simulink model "mod3tb_CIFF_CRFF_1bit"  (Simulink 7.9)
settings: Solver=VariableStepDiscrete  StartTime=0.0  StopTime=simu.trantime  RelTol=1e-3
undefined symbols (not defined in the file): a, b, c, Fs, g, mod
libraries: dspsigops x3, dspsrcs4 x1
settings Model: Creator=amyles  LastModifiedBy=Arnaldi Isacco
settings DataIOCC: MaxDataPoints=50000
settings OptimizationCC: InlineParams=on
settings DebuggingCC: UnderspecifiedInitializationDetection=Simplified  InvalidFcnCallConnMsg=none  StrictBusMsg=ErrorOnBusTreatedAsVector
settings ModelReferenceCC: ModelReferenceNumInstancesAllowed=Single
settings CodeAppCC: CustomSymbolStrType=$N$R$M_T
settings GRTTargetCC: CombineOutputUpdateFcns=off  GRTInterface=on

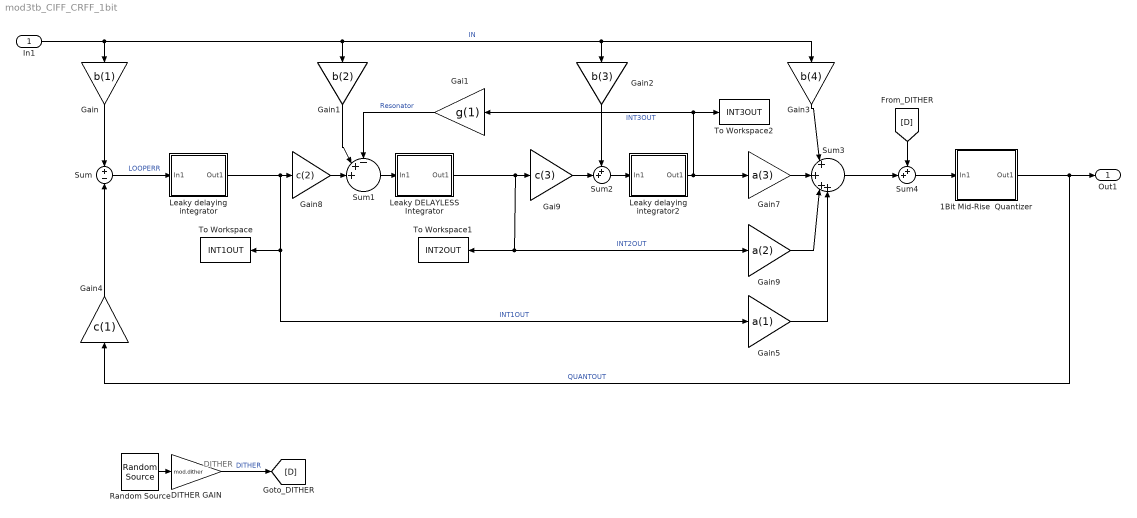
== system mod3tb_CIFF_CRFF_1bit ==
  note: DITHER
  In1 : Inport
  1Bit Mid-Rise  Quantizer : Subsystem
  DITHER GAIN : Gain  Gain=mod.dither  SampleTime=1/Fs
  Gai1 : Gain  Gain=g(1)
  Gai9 : Gain  Gain=c(3)
  Gain : Gain  Gain=b(1)
  Gain1 : Gain  Gain=b(2)
  Gain2 : Gain  Gain=b(3)
  Gain3 : Gain  Gain=b(4)
  Gain4 : Gain  Gain=c(1)
  Gain5 : Gain  Gain=a(1)
  Gain7 : Gain  Gain=a(3)
  Gain8 : Gain  Gain=c(2)
  Gain9 : Gain  Gain=a(2)
  Leaky DELAYLESS Integrator : Subsystem
  Leaky delaying integrator : Subsystem
  Leaky delaying integrator2 : Subsystem
  Random Source : dspsrcs4/Random Source  SrcType=Uniform  NormMethod=Ziggurat  CltLength=12  MinVal=-1  MaxVal=1  MeanVal=0  VarVal=1  RepMode=Not repeatable  rawSeed=1  IsInherit=off  SampMode=Discrete  SampTime=1/Fs  SampFrame=1  DataType=Double  OutComplex=Real
  Sum : Sum  Inputs=+-  SampleTime=1/Fs
  Sum1 : Sum  Inputs=-++||  SampleTime=1/Fs
  Sum2 : Sum  Inputs=++|  SampleTime=1/Fs
  Sum3 : Sum  Inputs=|+|+|++  SampleTime=1/Fs
  Sum4 : Sum  Inputs=++|
  To Workspace : ToWorkspace  VariableName=INT1OUT  SampleTime=-1
  To Workspace1 : ToWorkspace  VariableName=INT2OUT  SampleTime=-1
  To Workspace2 : ToWorkspace  VariableName=INT3OUT  SampleTime=-1
  Out1 : Outport
  wires:
  In1/1 -> Gain3/1, Gain2/1, Gain1/1, Gain/1  "IN"
  Gain8/1 -> Sum1/3
  Leaky DELAYLESS Integrator/1(Out1) -> Gai9/1, Gain9/1, To Workspace1/1  "INT2OUT"
  Gai9/1 -> Sum2/2
  Leaky delaying integrator2/1(Out1) -> Gain7/1, To Workspace2/1, Gai1/1  "INT3OUT"
  Gain4/1 -> Sum/2
  Gain/1 -> Sum/1
  Gain1/1 -> Sum1/2
  Gai1/1 -> Sum1/1  "Resonator"
  Gain2/1 -> Sum2/1
  1Bit Mid-Rise  Quantizer/1(Out1) -> Out1/1, Gain4/1  "QUANTOUT"
  Sum/1 -> Leaky delaying integrator/1(In1)  "LOOPERR"
  Sum2/1 -> Leaky delaying integrator2/1(In1)
  Sum1/1 -> Leaky DELAYLESS Integrator/1(In1)
  Gain3/1 -> Sum3/1
  Gain7/1 -> Sum3/2
  Gain9/1 -> Sum3/3
  Gain5/1 -> Sum3/4
  Random Source/1 -> DITHER GAIN/1
  DITHER GAIN/1 -> [D]  "DITHER"
  Leaky delaying integrator/1(Out1) -> Gain8/1, Gain5/1, To Workspace/1  "INT1OUT"
  [D] -> Sum4/1
  Sum3/1 -> Sum4/2
  Sum4/1 -> 1Bit Mid-Rise  Quantizer/1(In1)

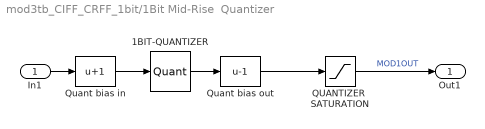
== system mod3tb_CIFF_CRFF_1bit/1Bit Mid-Rise  Quantizer ==
  In1 : Inport
  1BIT-QUANTIZER : Quantizer  QuantizationInterval=2  LinearizeAsGain=off  SampleTime=1/Fs
      settings: AttributesFormatString=step = 2
  QUANTIZER  SATURATION : Saturate  UpperLimit=mod.qsatout1  LowerLimit=-(mod.qsatout1)
      settings: AttributesFormatString=Limit quantizer\noutput
  Quant bias in : Bias  Bias=1
      settings: AttributesFormatString=Need offset to give\nMID-RISE quantiser
  Quant bias out : Bias  Bias=-1
      settings: AttributesFormatString=Shift outputs to\n..., -2, 1, 1, ...
  Out1 : Outport
  wires:
  Quant bias out/1 -> QUANTIZER  SATURATION/1
  Quant bias in/1 -> 1BIT-QUANTIZER/1
  1BIT-QUANTIZER/1 -> Quant bias out/1
  QUANTIZER  SATURATION/1 -> Out1/1  "MOD1OUT"
  In1/1 -> Quant bias in/1

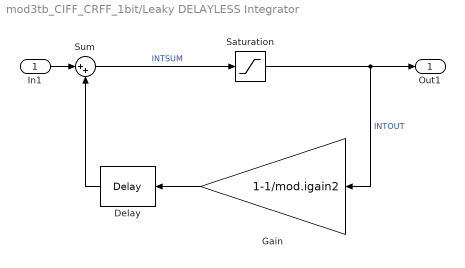
== system mod3tb_CIFF_CRFF_1bit/Leaky DELAYLESS Integrator ==
  In1 : Inport
  Delay : dspsigops/Delay  InputProcessing=Inherited (this choice will be removed - see release notes)  dly_unit=Samples  delay=1  ic_detail=off  dif_ic_for_ch=off  dif_ic_for_dly=off  ic=0  reset_popup=None
  Gain : Gain  Gain=1-1/mod.igain2
      settings: AttributesFormatString=Integrator leakage
  Saturation : Saturate  UpperLimit=mod.isat2  LowerLimit=-(mod.isat2)
  Sum : Sum  Inputs=|++
      settings: AttributesFormatString=Integrator summer
  Out1 : Outport
  wires:
  In1/1 -> Sum/1
  Saturation/1 -> Out1/1, Gain/1  "INTOUT"
  Gain/1 -> Delay/1
  Sum/1 -> Saturation/1  "INTSUM"
  Delay/1 -> Sum/2

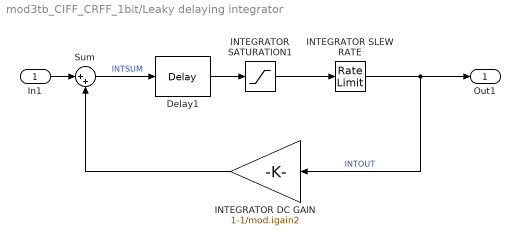
== system mod3tb_CIFF_CRFF_1bit/Leaky delaying integrator ==
  In1 : Inport
  Delay1 : dspsigops/Delay  InputProcessing=Inherited (this choice will be removed - see release notes)  dly_unit=Samples  delay=1  ic_detail=off  dif_ic_for_ch=off  dif_ic_for_dly=off  ic=0  reset_popup=None
  INTEGRATOR SATURATION1 : Saturate  UpperLimit=mod.isat2  LowerLimit=-(mod.isat2)
  INTEGRATOR SLEW RATE : RateLimiter  RisingSlewLimit=mod.isr1  FallingSlewLimit=-(mod.isr1)  SampleTimeMode=inherited
  INTEGRATOR DC GAIN : Gain  Gain=1-1/mod.igain2
      settings: AttributesFormatString=Integrator leakage\n(model finite integrator dc/LF\ngain in analog modulators)
  Sum : Sum  Inputs=|++
      settings: AttributesFormatString=Integrator summer
  Out1 : Outport
  wires:
  Sum/1 -> Delay1/1  "INTSUM"
  INTEGRATOR DC GAIN/1 -> Sum/2
  INTEGRATOR SATURATION1/1 -> INTEGRATOR SLEW RATE/1
  In1/1 -> Sum/1
  Delay1/1 -> INTEGRATOR SATURATION1/1
  INTEGRATOR SLEW RATE/1 -> Out1/1, INTEGRATOR DC GAIN/1  "INTOUT"

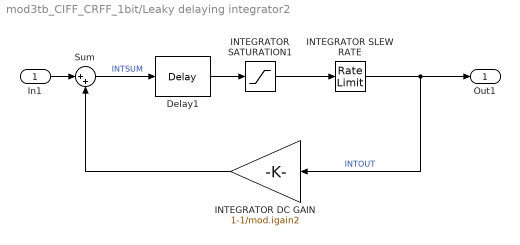
== system mod3tb_CIFF_CRFF_1bit/Leaky delaying integrator2 ==
  In1 : Inport
  Delay1 : dspsigops/Delay  InputProcessing=Inherited (this choice will be removed - see release notes)  dly_unit=Samples  delay=1  ic_detail=off  dif_ic_for_ch=off  dif_ic_for_dly=off  ic=0  reset_popup=None
  INTEGRATOR SATURATION1 : Saturate  UpperLimit=mod.isat2  LowerLimit=-(mod.isat2)
  INTEGRATOR SLEW RATE : RateLimiter  RisingSlewLimit=mod.isr1  FallingSlewLimit=-(mod.isr1)  SampleTimeMode=inherited
  INTEGRATOR DC GAIN : Gain  Gain=1-1/mod.igain2
      settings: AttributesFormatString=Integrator leakage\n(model finite integrator dc/LF\ngain in analog modulators)
  Sum : Sum  Inputs=|++
      settings: AttributesFormatString=Integrator summer
  Out1 : Outport
  wires:
  Sum/1 -> Delay1/1  "INTSUM"
  INTEGRATOR DC GAIN/1 -> Sum/2
  INTEGRATOR SATURATION1/1 -> INTEGRATOR SLEW RATE/1
  In1/1 -> Sum/1
  Delay1/1 -> INTEGRATOR SATURATION1/1
  INTEGRATOR SLEW RATE/1 -> Out1/1, INTEGRATOR DC GAIN/1  "INTOUT"
